simulink library "rfsoc_hdl_utils"  (R2019b)
settings: Solver=VariableStepAuto  StartTime=0.0  StopTime=10.0  RelTol=1e-3
libraries: simulink x3, hdlsllib x1
settings Model: Creator=tmealey  LastModifiedBy=tmealey
settings SFSimCC: CustomCodeUndefinedFunction=UseInterfaceOnly

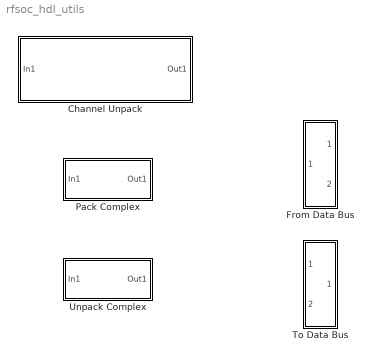
== system rfsoc_hdl_utils ==
  Channel Unpack : Subsystem  mask(Channel Unpack){samplesPerClock=4, complexSamples=on, reqBitWidth=0}
      mask prompts: samplesPerClock "Samples per clock"; complexSamples "Complex Samples"
      mask help:
      | Unpacks concatenated M vector samples DataIn into DataOut vector of  size [M, 1].
      |
      | If Complex Samples is true, assumes that I and Q are interleaved so that DataIn is of length M*bitsPerSample*2. Otherwise DataIn is of length M*bitsPersample.
      mask init:
      | if complexSamples
      |     input_length = samplesPerClock*2;
      | else
      |     input_length = samplesPerClock;
      | end
      | reqBitWidth = input_length*16;
      mask Display:
      | if complexSamples
      |     BitWidth = samplesPerClock*2*16;
      |     msg_bottom = 'Complex';
      |     label_out = sprintf('[%dx16-bit]',samplesPerClock);
      | else
      |     BitWidth = samplesPerClock*16;
      |     msg_bottom = 'Real';
      |     label_out = sprintf('[%dx16-bit]',samplesPerClock);
      | 
      | end
      | 
      | ReqBitWidth =  num2str(BitWidth);
      | fprintf('Channel \n Unpack')
      | %text(0.50, 0.50, 'AXI4 Read', 'horizontalAlignment', 'center');
      | %color('blue');
      | %text(0.97, 0.87,'ALTERASOC', 'horizontalAlignment', 'right');
      | 
      | label_in = sprintf('[%d-bit]',BitWidth);
      | 
      | port_label('input',1,sprintf('DataIn \n%s',label_in))
      | port_label('output',1,sprintf('DataOut \n%s',label_out))
      | 
      | 
      | color('red');
      | text(0.98, 0.15, msg_bottom, 'horizontalAlignment', 'right')
  From Data Bus : Subsystem  mask(From Data Bus){dummy=0}
      mask help: Convert a streaming Data Bus to individual Data and Valid signals.
      mask Display:
      | port_label('output',1,'data');
      | port_label('output',2,'valid');
  Pack Complex : Subsystem  mask(Pack Complex){dummy=0}
      mask help:
      | Convert complex value to packed word.
      |
      | Real component goes to lower bits; imaginary component goes to upper bits.
      mask Display: fprintf('Pack\nComplex');
  To Data Bus : Subsystem  mask(To Data Bus){dummy=0}
      mask help: Create a streaming Data Bus from Data and Valid signals.
      mask Display:
      | port_label('input',1,'data');
      | port_label('input',2,'valid');
  Unpack Complex : Subsystem  mask(Convert packed word to complex value.){datatype=fixdt(1,16,0)}
      mask prompts: datatype "Output datatype:"
      mask help: Real component extracted from lower bits; imaginary component extracted from upper bits.
      mask Display: fprintf('Unpack\nComplex');

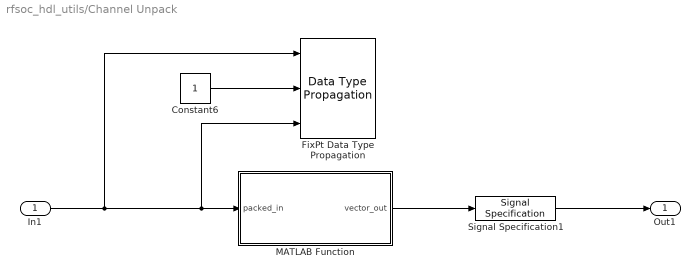
== system rfsoc_hdl_utils/Channel Unpack ==
  In1 : Inport
  Constant6 : Constant  OutDataTypeStr=int16  SampleTime=-1
  FixPt Data Type Propagation : simulink/Signal Attributes/Data Type Propagation  PropDataType=sfix(16)  IfRefDouble=double  IfRefSingle=single  IsSigned=IsSigned1  NumBitsBase=NumBits1  NumBitsMult=1  NumBitsAdd=0  NumBitsAllowFinal=reqBitWidth  PropScaling=2^-10  ValuesUsedBestPrec=[5 -7]  SlopeBase=Slope1  SlopeMult=1  SlopeAdd=0  BiasBase=Bias1  BiasMult=1  BiasAdd=0
      settings: SourceProductName=Simulink  SourceProductBaseCode=SL
  MATLAB Function : MATLAB Function  TreatAsAtomicUnit=on
  Signal Specification1 : SignalSpecification  Dimensions=[samplesPerClock 1]
  Out1 : Outport  VectorParamsAs1DForOutWhenUnconnected=off
  wires:
  MATLAB Function/1(vector_out) -> Signal Specification1/1
  Constant6/1 -> FixPt Data Type Propagation/2
  In1/1 -> FixPt Data Type Propagation/1, FixPt Data Type Propagation/3, MATLAB Function/1(packed_in)
  Signal Specification1/1 -> Out1/1

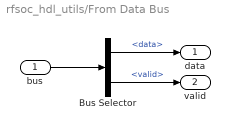
== system rfsoc_hdl_utils/From Data Bus ==
  bus : Inport
  Bus Selector : BusSelector  OutputSignals=data,valid
  data : Outport  VectorParamsAs1DForOutWhenUnconnected=off
  valid : Outport  Port=2  VectorParamsAs1DForOutWhenUnconnected=off
  wires:
  Bus Selector/2 -> valid/1  "<valid>"
  Bus Selector/1 -> data/1  "<data>"
  bus/1 -> Bus Selector/1

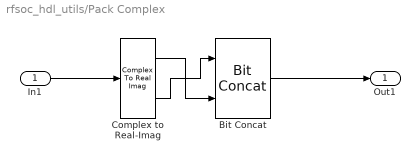
== system rfsoc_hdl_utils/Pack Complex ==
  In1 : Inport
  Bit Concat : hdlsllib/Logic and Bit Operations/Bit Concat  numInputs=2
      settings: SourceProductName=HDL Coder  SourceProductBaseCode=HD
  Complex to Real-Imag : ComplexToRealImag
  Out1 : Outport  VectorParamsAs1DForOutWhenUnconnected=off
  wires:
  Complex to Real-Imag/2 -> Bit Concat/1
  Complex to Real-Imag/1 -> Bit Concat/2
  Bit Concat/1 -> Out1/1
  In1/1 -> Complex to Real-Imag/1

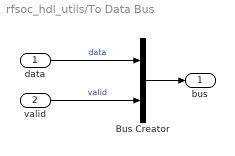
== system rfsoc_hdl_utils/To Data Bus ==
  data : Inport
  valid : Inport  Port=2
  Bus Creator : BusCreator  Inputs=2
  bus : Outport  VectorParamsAs1DForOutWhenUnconnected=off
  wires:
  Bus Creator/1 -> bus/1
  data/1 -> Bus Creator/1  "data"
  valid/1 -> Bus Creator/2  "valid"

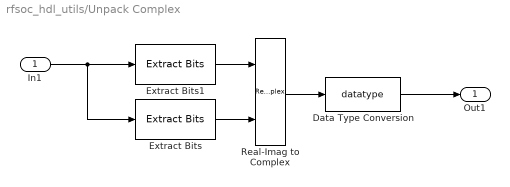
== system rfsoc_hdl_utils/Unpack Complex ==
  In1 : Inport
  Data Type Conversion : DataTypeConversion  OutDataTypeStr=datatype  ConvertRealWorld=Stored Integer (SI)
  Extract Bits : simulink/Logic and Bit Operations/Extract Bits  bitsToExtract=Upper half  numBits=8  bitIdxRange=[0 7]  outScalingMode=Treat bit field as an integer
      settings: SourceProductName=Simulink
  Extract Bits1 : simulink/Logic and Bit Operations/Extract Bits  bitsToExtract=Lower half  numBits=8  bitIdxRange=[0 7]  outScalingMode=Treat bit field as an integer
      settings: SourceProductName=Simulink
  Real-Imag to Complex : RealImagToComplex
  Out1 : Outport  VectorParamsAs1DForOutWhenUnconnected=off
  wires:
  Extract Bits/1 -> Real-Imag to Complex/2
  Extract Bits1/1 -> Real-Imag to Complex/1
  Data Type Conversion/1 -> Out1/1
  Real-Imag to Complex/1 -> Data Type Conversion/1
  In1/1 -> Extract Bits1/1, Extract Bits/1

== matlab function rfsoc_hdl_utils/Channel Unpack/MATLAB Function ==
  data: packed_in input; vector_out output; samplesPerClock parameter; complexSamples parameter
function vector_out = fcn(packed_in, samplesPerClock, complexSamples)
%#codegen
%
% unpacks incoming ufixN packed_in into vector_out ([samplesPerClock, 1])
% assumes that samplesPerClock samples are packed into the input
% if complexSamples is true, assumes that I and Q are interleaved so that 
% packed_in is of length samplesPerClock*bitsPerSample*2. Otherwise
% packed_in is of length samplesPerClock*bitsPersample
%
% Greg Ushomirsky, Systems & Technology Research, 2019.
bitsPerSample = 16;

if complexSamples
    inputLength = coder.const(samplesPerClock*2);
else
    inputLength = coder.const(samplesPerClock);
end

packed_in_fi = cast_to_fi(packed_in);

unpacked_out = zeros(inputLength,1,'like',fi(0,1,bitsPerSample,0));
% elem = int64(0);

% need to unroll this loop at compile time because bitsliceget requires 
% constant inputs 
coder.unroll(); 
for n=1:inputLength
    rightIdx = (n-1)*bitsPerSample + 1;
    leftIdx  = n*bitsPerSample;
    elem =  bitsliceget(packed_in_fi,leftIdx,rightIdx);
    unpacked_out(n) = reinterpretcast(elem, numerictype(1,bitsPerSample,0));
end

if complexSamples
    vector_out = complex(unpacked_out(1:2:end),unpacked_out(2:2:end));
else
    vector_out = unpacked_out;
end
